simulink model "ACC_Controller_MIL"  (R2015a)
settings: Solver=FixedStepDiscrete  StartTime=0.0  StopTime=20.0  RelTol=1e-3
undefined symbols (not defined in the file): D_clear, D_min, Kp_dist, Kp_spd, Kv_rel, sigbuilder_block, T_gap, T_max, T_min
settings Model: Creator=A.hegazy  LastModifiedBy=A.hegazy
settings OptimizationCC: OptimizeModelRefInitCode=on  LifeSpan=1
settings RTWCC: SystemTargetFile=ert.tlc  TemplateMakefile=ert_default_tmf  Description=Embedded Coder
settings CodeAppCC: IgnoreCustomStorageClasses=off
settings ERTTargetCC: ParMdlRefBuildCompliant=on  CompOptLevelCompliant=on  ConcurrentExecutionCompliant=on  ERTFirstTimeCompliant=on  SupportContinuousTime=off  SupportVariableSizeSignals=off  ModelStepFunctionPrototypeControlCompliant=on  CPPClassGenCompliant=on  InlinedParameterPlacement=Hierarchical  ERTCustomFileTemplate=example_file_process.tlc

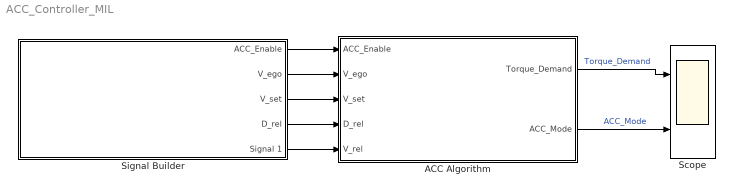
== system ACC_Controller_MIL ==
  ACC Algorithm : Subsystem
  Scope : Scope  NumInputPorts=2
      settings: YMin=-5~-5  YMax=5~5
  Signal Builder : Subsystem  Tag=STV Subsys  LoadFcn=sigbuilder_block('load');  StartFcn=sigbuilder_block('start');  StopFcn=sigbuilder_block('stop');  ClipboardFcn=sigbuilder_block('clipboard');  mask(Sigbuilder block){}
      mask help: Simulink:masks:SigbuilderBlock_MD
      mask init:
      | if ~strcmp(get_param(bdroot(gcbh),'SimulationStatus'),'stopped') tuvar = sigbuilder_block('maskInit'); end
      settings: CopyFcn=sigbuilder_block('copy');  DeleteFcn=sigbuilder_block('delete');  ModelCloseFcn=sigbuilder_block('modelClose');  PreSaveFcn=sigbuilder_block('preSave');  PauseFcn=sigbuilder_block('pause');  ContinueFcn=sigbuilder_block('continue');  NameChangeFcn=sigbuilder_block('namechange');  OpenFcn=sigbuilder_block('open',[437.6 199.2 550.4 400 ]);  CloseFcn=sigbuilder_block('close');
      mask Display: plot(0, 0, 100, 100,[2, 2, 32, 32, 2], [68, 8, 8, 68, 68],[32, 2], [38, 38], [32, 19, 2],[53, 60, 44], [32, 17, 17, 2],[16, 16, 31, 31]);txt = getActiveGroup(gcbh);text(2, 100, txt,'verticalAlignment', 'top');
  wires:
  ACC Algorithm/1(Torque_Demand) -> Scope/1  "Torque_Demand"
  ACC Algorithm/2(ACC_Mode) -> Scope/2  "ACC_Mode"
  Signal Builder/1(ACC_Enable) -> ACC Algorithm/1(ACC_Enable)
  Signal Builder/2(V_ego) -> ACC Algorithm/2(V_ego)
  Signal Builder/3(V_set) -> ACC Algorithm/3(V_set)
  Signal Builder/4(D_rel) -> ACC Algorithm/4(D_rel)
  Signal Builder/5(Signal 1) -> ACC Algorithm/5(V_rel)

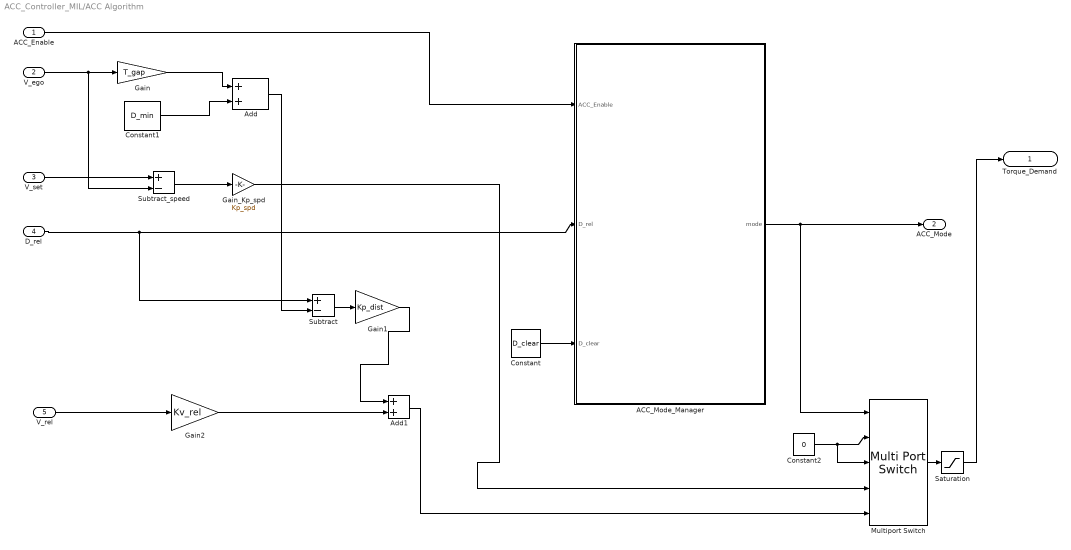
== system ACC_Controller_MIL/ACC Algorithm ==
  ACC_Enable : Inport
  V_ego : Inport  Port=2
  V_set : Inport  Port=3
  D_rel : Inport  Port=4
  V_rel : Inport  Port=5
  ACC_Mode_Manager : Stateflow chart  TreatAsAtomicUnit=on
  Add : Sum
  Add1 : Sum
  Constant : Constant  Value=D_clear
  Constant1 : Constant  Value=D_min
  Constant2 : Constant  Value=0
  Gain : Gain  Gain=T_gap
  Gain1 : Gain  Gain=Kp_dist
  Gain2 : Gain  Gain=Kv_rel
  Gain_Kp_spd : Gain  Gain=Kp_spd
  Multiport Switch : MultiPortSwitch  DataPortOrder=Zero-based contiguous  Inputs=4  DiagnosticForDefault=None
  Saturation : Saturate  UpperLimit=T_max  LowerLimit=T_min
  Subtract : Sum  Inputs=+-
  Subtract_speed : Sum  Inputs=+-
  Torque_Demand : Outport
  ACC_Mode : Outport  Port=2
  wires:
  ACC_Enable/1 -> ACC_Mode_Manager/1(ACC_Enable)
  D_rel/1 -> ACC_Mode_Manager/2(D_rel), Subtract/1
  Constant/1 -> ACC_Mode_Manager/3(D_clear)
  V_ego/1 -> Subtract_speed/2, Gain/1
  Gain/1 -> Add/1
  Constant1/1 -> Add/2
  Add/1 -> Subtract/2
  Subtract/1 -> Gain1/1
  V_rel/1 -> Gain2/1
  Gain1/1 -> Add1/1
  Gain2/1 -> Add1/2
  V_set/1 -> Subtract_speed/1
  Subtract_speed/1 -> Gain_Kp_spd/1
  Gain_Kp_spd/1 -> Multiport Switch/4
  Add1/1 -> Multiport Switch/5
  ACC_Mode_Manager/1(mode) -> Multiport Switch/1, ACC_Mode/1
  Multiport Switch/1 -> Saturation/1
  Saturation/1 -> Torque_Demand/1
  Constant2/1 -> Multiport Switch/3, Multiport Switch/2

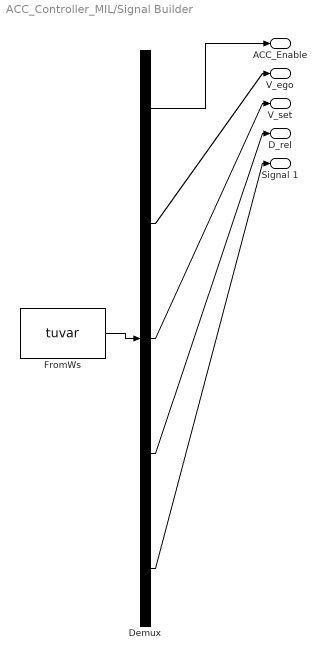
== system ACC_Controller_MIL/Signal Builder ==
  Demux : Demux  Tag=STV Demux  Outputs=5
  FromWs : FromWorkspace  Tag=STV FromWs  VariableName=tuvar  SampleTime=0
      SigBuilderData=|
      | common.afterFinalStr = 'Extrapolate'
      | common.sampleTime = 0
      | dataSet.timeRange = [0 10]
      | dataSet.name = 'Group 1'
      | sbobj.Groups.Name = 'Group 1'
      | sbobj.Groups.Signals(1).Name = 'ACC_Enable'
      | sbobj.Groups.Signals(1).XData = [0 2 2 10]
      | sbobj.Groups.Signals(1).YData = [0 0 1 1]
      | sbobj.Groups.Signals(2).Name = 'V_ego'
      | sbobj.Groups.Signals(2).XData = [0 2 5 10]
      | sbobj.Groups.Signals(2).YData = [0 20 25 25]
      | sbobj.Groups.Signals(3).Name = 'V_set'
      | sbobj.Groups.Signals(3).XData = [0 10]
      | sbobj.Groups.Signals(3).YData = [30 30]
      | sbobj.Groups.Signals(4).Name = 'D_rel'
      | sbobj.Groups.Signals(4).XData = [0 5 5 10]
      | sbobj.Groups.Signals(4).YData = [100 100 30 30]
      | sbobj.Groups.Signals(5).Name = 'Signal 1'
      | sbobj.Groups.Signals(5).XData = [0 5 5 10]
      | sbobj.Groups.Signals(5).YData = [0 0 -5 -5]
  ACC_Enable : Outport  Tag=STV Outport
  V_ego : Outport  Tag=STV Outport  Port=2
  V_set : Outport  Tag=STV Outport  Port=3
  D_rel : Outport  Tag=STV Outport  Port=4
  Signal 1 : Outport  Tag=STV Outport  Port=5
  wires:
  Demux/1 -> ACC_Enable/1
  FromWs/1 -> Demux/1
  Demux/2 -> V_ego/1
  Demux/3 -> V_set/1
  Demux/4 -> D_rel/1
  Demux/5 -> Signal 1/1

== stateflow chart ACC_Controller_MIL/ACC Algorithm/ACC_Mode_Manager ==
  state Off
    entry: mode = 0;
  state Standby
    entry: mode = 1;
  state Distance_Control
    entry: mode= 3;
  state Speed_Control
    entry: mode= 2;
  (default) -> Off
  Distance_Control -> Off [order 2] : [ACC_Enable == 0]
  Speed_Control -> Off [order 2] : [ACC_Enable == 0]
  Standby -> Off [order 1] : [ACC_Enable == 0]
  Off -> Standby : [ACC_Enable == 1]
  Standby -> Speed_Control [order 2] : [ACC_Enable == 1 && D_rel > D_clear]
  Standby -> Distance_Control [order 3] : [ACC_Enable == 1 && D_rel <= D_clear]
  Distance_Control -> Speed_Control [order 1] : [D_rel > D_clear]
  Speed_Control -> Distance_Control [order 1] : [D_rel <= D_clear]
  data: ACC_Enable input; D_rel input; D_clear input; mode output
